simulink model "flc"  (R2019b)
settings: Solver=VariableStepAuto  StartTime=0.0  StopTime=10.0  RelTol=1e-3
undefined symbols (not defined in the file): Ts
libraries: fuzblock x1
settings Model: Creator=hermankj  LastModifiedBy=hermankj

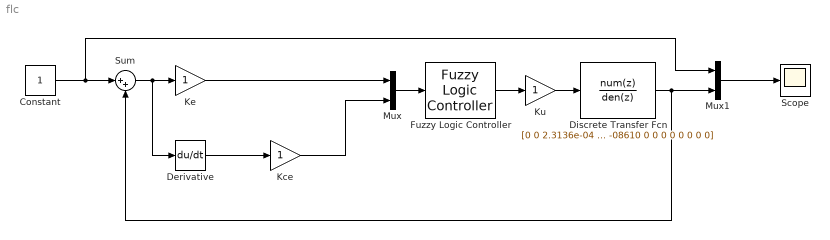
== system flc ==
  Constant : Constant
  Derivative : Derivative
  Discrete Transfer Fcn : DiscreteTransferFcn  Numerator=[0 0 2.3136e-04 9.2800e-07 0 0 0 0 0 0 0 0]  Denominator=[1 -2.8560 2.7170 -08610 0 0 0 0 0 0 0 0]  SampleTime=Ts
  Fuzzy Logic Controller : fuzblock/Fuzzy Logic  Controller  FIS='tipper.fis'  OutputSampleNumber=101  DataType=double  FuzzifiedInputs=off  RuleFiringStrengths=off  RuleOutputs=off  AggregatedOutputs=off  SimulateUsing=Interpreted execution  OutOfRangeInputValueMessage=warning  NoRuleFiredMessage=warning  EmptyOutputFuzzySetMessage=warning
  "Kce " : Gain
  Ke : Gain
  "Ku " : Gain
  Mux : Mux  Inputs=2
  Mux1 : Mux  Inputs=2
  Scope : Scope
  Sum : Sum  Inputs=|++
  wires:
  Constant/1 -> Mux1/1, Sum/1
  Sum/1 -> Derivative/1, Ke/1
  Derivative/1 -> "Kce "/1
  Ke/1 -> Mux/1
  "Kce "/1 -> Mux/2
  Mux/1 -> Fuzzy Logic Controller/1
  Fuzzy Logic Controller/1 -> "Ku "/1
  Mux1/1 -> Scope/1
  "Ku "/1 -> Discrete Transfer Fcn/1
  Discrete Transfer Fcn/1 -> Sum/2, Mux1/2
